simulink model "TEST_IPM_CPU2"  (R2019b)
settings: configuration reference "Configuration_CPU2" (kept outside this file)
libraries: c2837xDlib x2, c2000lib x1
settings Model: DataDictionary=TEST_IPM_LIB.sldd  Creator=Downstream  LastModifiedBy=Downstream
settings ConfigSetRef: SourceName=Configuration_CPU2

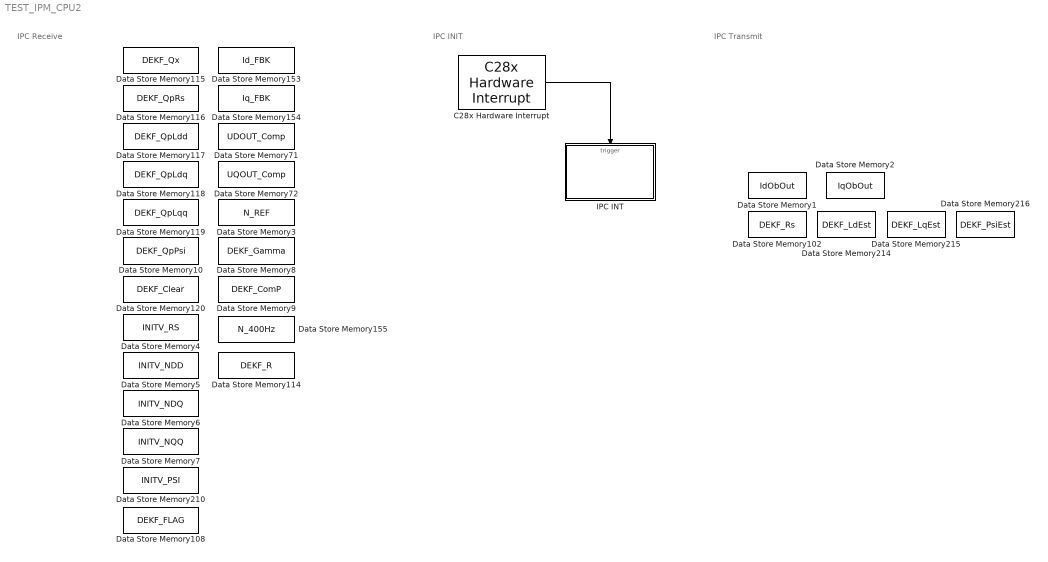
== system TEST_IPM_CPU2 ==
  note: IPC INIT
  note: IPC Receive
  note: IPC Transmit
  C28x Hardware Interrupt : c2000lib/Scheduling/C28x Hardware Interrupt  irqnumbers=[1]  pienumbers=[13]  irqpriorities=[4]  irqpreempts=[0]  showinput=off  dspchiptype=C280X
      settings: SourceProductName=Embedded Coder Support Package for Texas Instruments C2000 Processors  SourceProductBaseCode=TIC2000
  Data Store Memory1 : DataStoreMemory  DataStoreName=IdObOut  ReadBeforeWriteMsg=warning  WriteAfterWriteMsg=warning  WriteAfterReadMsg=warning  ShowAdditionalParam=off  OutDataTypeStr=single
      settings: RTWStateStorageClass=ExportedGlobal
  Data Store Memory10 : DataStoreMemory  DataStoreName=DEKF_QpPsi  ReadBeforeWriteMsg=warning  WriteAfterWriteMsg=warning  WriteAfterReadMsg=warning  InitialValue=0.047  ShowAdditionalParam=off  OutDataTypeStr=single
      settings: RTWStateStorageClass=ExportedGlobal
  Data Store Memory102 : DataStoreMemory  DataStoreName=DEKF_Rs  ReadBeforeWriteMsg=warning  WriteAfterWriteMsg=warning  WriteAfterReadMsg=warning  ShowAdditionalParam=off  OutDataTypeStr=single
      settings: RTWStateStorageClass=ExportedGlobal
  Data Store Memory108 : DataStoreMemory  DataStoreName=DEKF_FLAG  ReadBeforeWriteMsg=warning  WriteAfterWriteMsg=warning  WriteAfterReadMsg=warning  ShowAdditionalParam=off  OutDataTypeStr=uint16
      settings: RTWStateStorageClass=ExportedGlobal
  Data Store Memory114 : DataStoreMemory  DataStoreName=DEKF_R  ReadBeforeWriteMsg=warning  WriteAfterWriteMsg=warning  WriteAfterReadMsg=warning  ShowAdditionalParam=off  OutDataTypeStr=single
      settings: RTWStateStorageClass=ExportedGlobal
  Data Store Memory115 : DataStoreMemory  DataStoreName=DEKF_Qx  ReadBeforeWriteMsg=warning  WriteAfterWriteMsg=warning  WriteAfterReadMsg=warning  ShowAdditionalParam=off  OutDataTypeStr=single
      settings: RTWStateStorageClass=ExportedGlobal
  Data Store Memory116 : DataStoreMemory  DataStoreName=DEKF_QpRs  ReadBeforeWriteMsg=warning  WriteAfterWriteMsg=warning  WriteAfterReadMsg=warning  ShowAdditionalParam=off  OutDataTypeStr=single
      settings: RTWStateStorageClass=ExportedGlobal
  Data Store Memory117 : DataStoreMemory  DataStoreName=DEKF_QpLdd  ReadBeforeWriteMsg=warning  WriteAfterWriteMsg=warning  WriteAfterReadMsg=warning  ShowAdditionalParam=off  OutDataTypeStr=single
      settings: RTWStateStorageClass=ExportedGlobal
  Data Store Memory118 : DataStoreMemory  DataStoreName=DEKF_QpLdq  ReadBeforeWriteMsg=warning  WriteAfterWriteMsg=warning  WriteAfterReadMsg=warning  ShowAdditionalParam=off  OutDataTypeStr=single
      settings: RTWStateStorageClass=ExportedGlobal
  Data Store Memory119 : DataStoreMemory  DataStoreName=DEKF_QpLqq  ReadBeforeWriteMsg=warning  WriteAfterWriteMsg=warning  WriteAfterReadMsg=warning  ShowAdditionalParam=off  OutDataTypeStr=single
      settings: RTWStateStorageClass=ExportedGlobal
  Data Store Memory120 : DataStoreMemory  DataStoreName=DEKF_Clear  ReadBeforeWriteMsg=warning  WriteAfterWriteMsg=warning  WriteAfterReadMsg=warning  ShowAdditionalParam=off  OutDataTypeStr=uint16
      settings: RTWStateStorageClass=ExportedGlobal
  Data Store Memory153 : DataStoreMemory  DataStoreName=Id_FBK  ReadBeforeWriteMsg=warning  WriteAfterWriteMsg=warning  WriteAfterReadMsg=warning  ShowAdditionalParam=off  OutDataTypeStr=single
      settings: RTWStateStorageClass=ExportedGlobal
  Data Store Memory154 : DataStoreMemory  DataStoreName=Iq_FBK  ReadBeforeWriteMsg=warning  WriteAfterWriteMsg=warning  WriteAfterReadMsg=warning  ShowAdditionalParam=off  OutDataTypeStr=single
      settings: RTWStateStorageClass=ExportedGlobal
  Data Store Memory155 : DataStoreMemory  DataStoreName=N_400Hz  ReadBeforeWriteMsg=warning  WriteAfterWriteMsg=warning  WriteAfterReadMsg=warning  ShowAdditionalParam=off  OutDataTypeStr=single
      settings: RTWStateStorageClass=ExportedGlobal
  Data Store Memory2 : DataStoreMemory  DataStoreName=IqObOut  ReadBeforeWriteMsg=warning  WriteAfterWriteMsg=warning  WriteAfterReadMsg=warning  ShowAdditionalParam=off  OutDataTypeStr=single
      settings: RTWStateStorageClass=ExportedGlobal
  Data Store Memory210 : DataStoreMemory  DataStoreName=INITV_PSI  ReadBeforeWriteMsg=warning  WriteAfterWriteMsg=warning  WriteAfterReadMsg=warning  InitialValue=0.047  ShowAdditionalParam=off  OutDataTypeStr=single
      settings: RTWStateStorageClass=ExportedGlobal
  Data Store Memory214 : DataStoreMemory  DataStoreName=DEKF_LdEst  ReadBeforeWriteMsg=warning  WriteAfterWriteMsg=warning  WriteAfterReadMsg=warning  ShowAdditionalParam=off  OutDataTypeStr=single
      settings: RTWStateStorageClass=ExportedGlobal
  Data Store Memory215 : DataStoreMemory  DataStoreName=DEKF_LqEst  ReadBeforeWriteMsg=warning  WriteAfterWriteMsg=warning  WriteAfterReadMsg=warning  ShowAdditionalParam=off  OutDataTypeStr=single
      settings: RTWStateStorageClass=ExportedGlobal
  Data Store Memory216 : DataStoreMemory  DataStoreName=DEKF_PsiEst  ReadBeforeWriteMsg=warning  WriteAfterWriteMsg=warning  WriteAfterReadMsg=warning  ShowAdditionalParam=off  OutDataTypeStr=single
      settings: RTWStateStorageClass=ExportedGlobal
  Data Store Memory3 : DataStoreMemory  DataStoreName=N_REF  ReadBeforeWriteMsg=warning  WriteAfterWriteMsg=warning  WriteAfterReadMsg=warning  ShowAdditionalParam=off  OutDataTypeStr=single
      settings: RTWStateStorageClass=ExportedGlobal
  Data Store Memory4 : DataStoreMemory  DataStoreName=INITV_RS  ReadBeforeWriteMsg=warning  WriteAfterWriteMsg=warning  WriteAfterReadMsg=warning  InitialValue=0.93  ShowAdditionalParam=off  OutDataTypeStr=single
      settings: RTWStateStorageClass=ExportedGlobal
  Data Store Memory5 : DataStoreMemory  DataStoreName=INITV_NDD  ReadBeforeWriteMsg=warning  WriteAfterWriteMsg=warning  WriteAfterReadMsg=warning  InitialValue=1/2.7e-3  ShowAdditionalParam=off  OutDataTypeStr=single
      settings: RTWStateStorageClass=ExportedGlobal
  Data Store Memory6 : DataStoreMemory  DataStoreName=INITV_NDQ  ReadBeforeWriteMsg=warning  WriteAfterWriteMsg=warning  WriteAfterReadMsg=warning  ShowAdditionalParam=off  OutDataTypeStr=single
      settings: RTWStateStorageClass=ExportedGlobal
  Data Store Memory7 : DataStoreMemory  DataStoreName=INITV_NQQ  ReadBeforeWriteMsg=warning  WriteAfterWriteMsg=warning  WriteAfterReadMsg=warning  InitialValue=1/4.9e-3  ShowAdditionalParam=off  OutDataTypeStr=single
      settings: RTWStateStorageClass=ExportedGlobal
  Data Store Memory71 : DataStoreMemory  DataStoreName=UDOUT_Comp  ReadBeforeWriteMsg=warning  WriteAfterWriteMsg=warning  WriteAfterReadMsg=warning  ShowAdditionalParam=off  OutDataTypeStr=single
      settings: RTWStateStorageClass=ExportedGlobal
  Data Store Memory72 : DataStoreMemory  DataStoreName=UQOUT_Comp  ReadBeforeWriteMsg=warning  WriteAfterWriteMsg=warning  WriteAfterReadMsg=warning  ShowAdditionalParam=off  OutDataTypeStr=single
      settings: RTWStateStorageClass=ExportedGlobal
  Data Store Memory8 : DataStoreMemory  DataStoreName=DEKF_Gamma  ReadBeforeWriteMsg=warning  WriteAfterWriteMsg=warning  WriteAfterReadMsg=warning  ShowAdditionalParam=off  OutDataTypeStr=single
      settings: RTWStateStorageClass=ExportedGlobal
  Data Store Memory9 : DataStoreMemory  DataStoreName=DEKF_ComP  ReadBeforeWriteMsg=warning  WriteAfterWriteMsg=warning  WriteAfterReadMsg=warning  ShowAdditionalParam=off  OutDataTypeStr=single
      settings: RTWStateStorageClass=ExportedGlobal
  IPC INT : Subsystem  TreatAsAtomicUnit=on
  wires:
  C28x Hardware Interrupt/1 -> IPC INT/Trigger

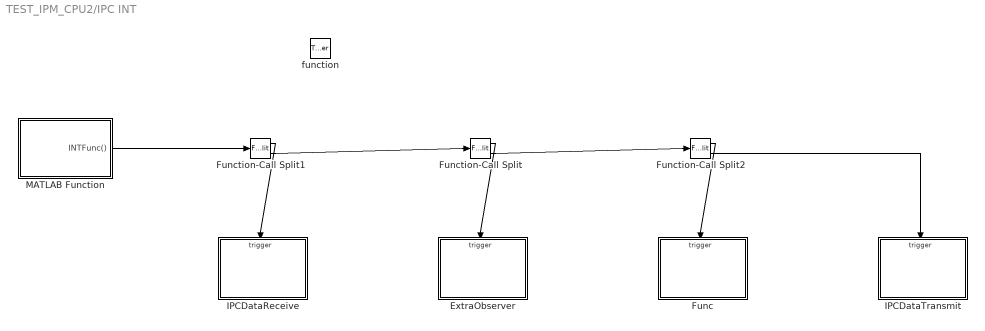
== system TEST_IPM_CPU2/IPC INT ==
  function : TriggerPort  TriggerType=function-call  VariantControl=Variant
  ExtraObserver : Subsystem
  Func : Subsystem
  Function-Call Split : FunctionCallSplit  NumOutputPorts=2
  Function-Call Split1 : FunctionCallSplit  NumOutputPorts=2
  Function-Call Split2 : FunctionCallSplit  NumOutputPorts=2
  IPCDataReceive : Subsystem
  IPCDataTransmit : Subsystem
  MATLAB Function : MATLAB Function  TreatAsAtomicUnit=on
  wires:
  MATLAB Function/1(INTFunc()) -> Function-Call Split1/1
  Function-Call Split1/1 -> IPCDataReceive/Trigger
  Function-Call Split/1 -> ExtraObserver/Trigger
  Function-Call Split1/2 -> Function-Call Split/1
  Function-Call Split/2 -> Function-Call Split2/1
  Function-Call Split2/2 -> IPCDataTransmit/Trigger
  Function-Call Split2/1 -> Func/Trigger

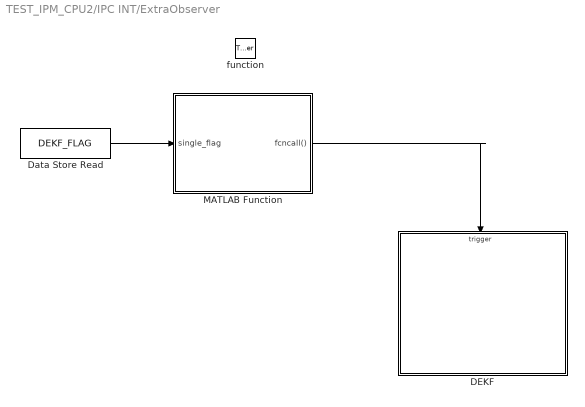
== system TEST_IPM_CPU2/IPC INT/ExtraObserver ==
  function : TriggerPort  TriggerType=function-call  VariantControl=Variant
  DEKF : Subsystem  TreatAsAtomicUnit=on
  Data Store Read : DataStoreRead  DataStoreName=DEKF_FLAG
  MATLAB Function : MATLAB Function  TreatAsAtomicUnit=on
  wires:
  Data Store Read/1 -> MATLAB Function/1(single_flag)
  MATLAB Function/1(fcncall()) -> DEKF/Trigger

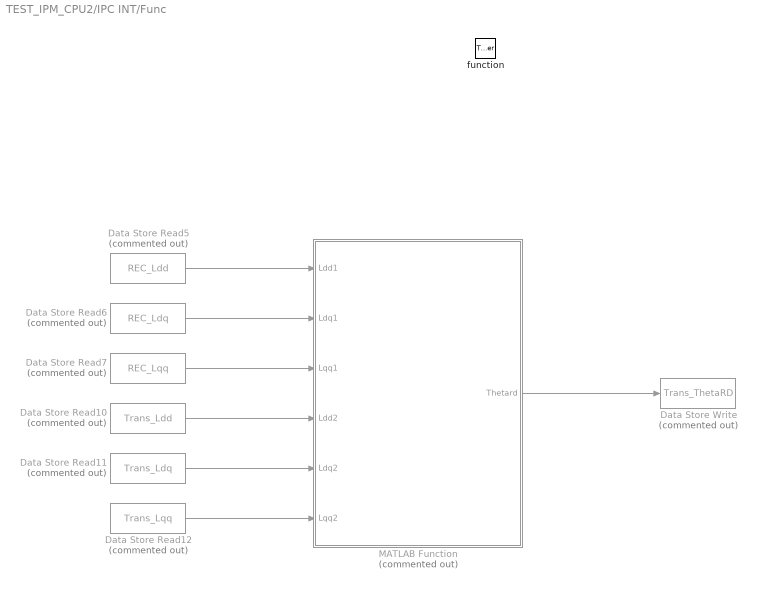
== system TEST_IPM_CPU2/IPC INT/Func ==
  function : TriggerPort  TriggerType=function-call  VariantControl=Variant
  Data Store Read10 : DataStoreRead  Commented=on  DataStoreName=Trans_Ldd
  Data Store Read11 : DataStoreRead  Commented=on  DataStoreName=Trans_Ldq
  Data Store Read12 : DataStoreRead  Commented=on  DataStoreName=Trans_Lqq
  Data Store Read5 : DataStoreRead  Commented=on  DataStoreName=REC_Ldd
  Data Store Read6 : DataStoreRead  Commented=on  DataStoreName=REC_Ldq
  Data Store Read7 : DataStoreRead  Commented=on  DataStoreName=REC_Lqq
  Data Store Write : DataStoreWrite  Commented=on  DataStoreName=Trans_ThetaRD
  MATLAB Function : MATLAB Function  Commented=on  TreatAsAtomicUnit=on
  wires:
  Data Store Read5/1 -> MATLAB Function/1(Ldd1)
  Data Store Read6/1 -> MATLAB Function/2(Ldq1)
  Data Store Read7/1 -> MATLAB Function/3(Lqq1)
  Data Store Read10/1 -> MATLAB Function/4(Ldd2)
  Data Store Read11/1 -> MATLAB Function/5(Ldq2)
  Data Store Read12/1 -> MATLAB Function/6(Lqq2)
  MATLAB Function/1(Thetard) -> Data Store Write/1

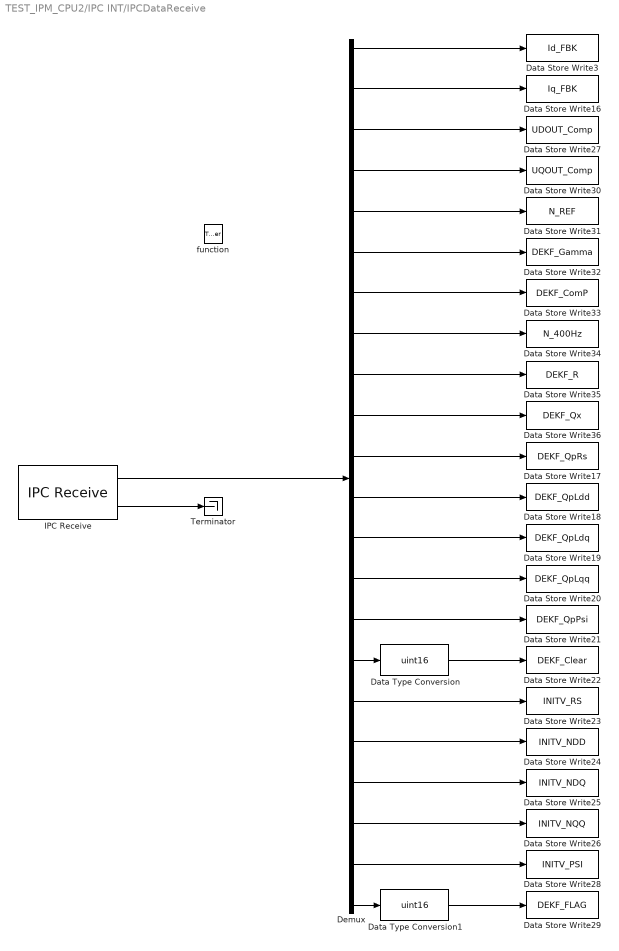
== system TEST_IPM_CPU2/IPC INT/IPCDataReceive ==
  function : TriggerPort  TriggerType=function-call  VariantControl=Variant
  Data Store Write16 : DataStoreWrite  DataStoreName=Iq_FBK
  Data Store Write17 : DataStoreWrite  DataStoreName=DEKF_QpRs
  Data Store Write18 : DataStoreWrite  DataStoreName=DEKF_QpLdd
  Data Store Write19 : DataStoreWrite  DataStoreName=DEKF_QpLdq
  Data Store Write20 : DataStoreWrite  DataStoreName=DEKF_QpLqq
  Data Store Write21 : DataStoreWrite  DataStoreName=DEKF_QpPsi
  Data Store Write22 : DataStoreWrite  DataStoreName=DEKF_Clear
  Data Store Write23 : DataStoreWrite  DataStoreName=INITV_RS
  Data Store Write24 : DataStoreWrite  DataStoreName=INITV_NDD
  Data Store Write25 : DataStoreWrite  DataStoreName=INITV_NDQ
  Data Store Write26 : DataStoreWrite  DataStoreName=INITV_NQQ
  Data Store Write27 : DataStoreWrite  DataStoreName=UDOUT_Comp
  Data Store Write28 : DataStoreWrite  DataStoreName=INITV_PSI
  Data Store Write29 : DataStoreWrite  DataStoreName=DEKF_FLAG
  Data Store Write3 : DataStoreWrite  DataStoreName=Id_FBK
  Data Store Write30 : DataStoreWrite  DataStoreName=UQOUT_Comp
  Data Store Write31 : DataStoreWrite  DataStoreName=N_REF
  Data Store Write32 : DataStoreWrite  DataStoreName=DEKF_Gamma
  Data Store Write33 : DataStoreWrite  DataStoreName=DEKF_ComP
  Data Store Write34 : DataStoreWrite  DataStoreName=N_400Hz
  Data Store Write35 : DataStoreWrite  DataStoreName=DEKF_R
  Data Store Write36 : DataStoreWrite  DataStoreName=DEKF_Qx
  Data Type Conversion : DataTypeConversion  OutDataTypeStr=uint16
  Data Type Conversion1 : DataTypeConversion  OutDataTypeStr=uint16
  Demux : Demux  Outputs=22
  IPC Receive : c2837xDlib/IPC Receive  SelectChannel=0  DataType=single  DataLength=22  EnableBlocking=off  SampleTime=-1
      settings: SourceProductName=Embedded Coder Support Package for Texas Instruments C2000 Processors  SourceProductBaseCode=TIC2000
  Terminator : Terminator
  wires:
  IPC Receive/1 -> Demux/1
  IPC Receive/2 -> Terminator/1
  Demux/1 -> Data Store Write3/1
  Demux/2 -> Data Store Write16/1
  Demux/3 -> Data Store Write27/1
  Demux/4 -> Data Store Write30/1
  Demux/5 -> Data Store Write31/1
  Demux/6 -> Data Store Write32/1
  Demux/7 -> Data Store Write33/1
  Demux/8 -> Data Store Write34/1
  Demux/9 -> Data Store Write35/1
  Demux/10 -> Data Store Write36/1
  Demux/11 -> Data Store Write17/1
  Demux/12 -> Data Store Write18/1
  Demux/13 -> Data Store Write19/1
  Demux/14 -> Data Store Write20/1
  Demux/15 -> Data Store Write21/1
  Demux/16 -> Data Type Conversion/1
  Demux/17 -> Data Store Write23/1
  Demux/18 -> Data Store Write24/1
  Demux/19 -> Data Store Write25/1
  Demux/20 -> Data Store Write26/1
  Demux/21 -> Data Store Write28/1
  Demux/22 -> Data Type Conversion1/1
  Data Type Conversion/1 -> Data Store Write22/1
  Data Type Conversion1/1 -> Data Store Write29/1

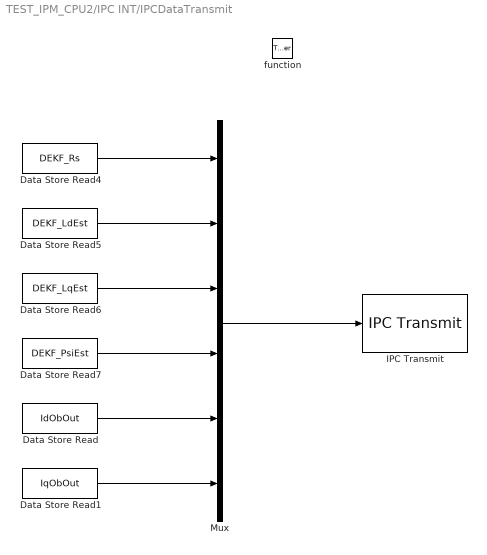
== system TEST_IPM_CPU2/IPC INT/IPCDataTransmit ==
  function : TriggerPort  TriggerType=function-call  VariantControl=Variant
  Data Store Read : DataStoreRead  DataStoreName=IdObOut
  Data Store Read1 : DataStoreRead  DataStoreName=IqObOut
  Data Store Read4 : DataStoreRead  DataStoreName=DEKF_Rs
  Data Store Read5 : DataStoreRead  DataStoreName=DEKF_LdEst
  Data Store Read6 : DataStoreRead  DataStoreName=DEKF_LqEst
  Data Store Read7 : DataStoreRead  DataStoreName=DEKF_PsiEst
  IPC Transmit : c2837xDlib/IPC Transmit  SelectChannel=1  EnableBlocking=off
      settings: SourceProductName=Embedded Coder Support Package for Texas Instruments C2000 Processors  SourceProductBaseCode=TIC2000
  Mux : Mux  Inputs=6
  wires:
  Mux/1 -> IPC Transmit/1
  Data Store Read4/1 -> Mux/1
  Data Store Read5/1 -> Mux/2
  Data Store Read6/1 -> Mux/3
  Data Store Read7/1 -> Mux/4
  Data Store Read/1 -> Mux/5
  Data Store Read1/1 -> Mux/6

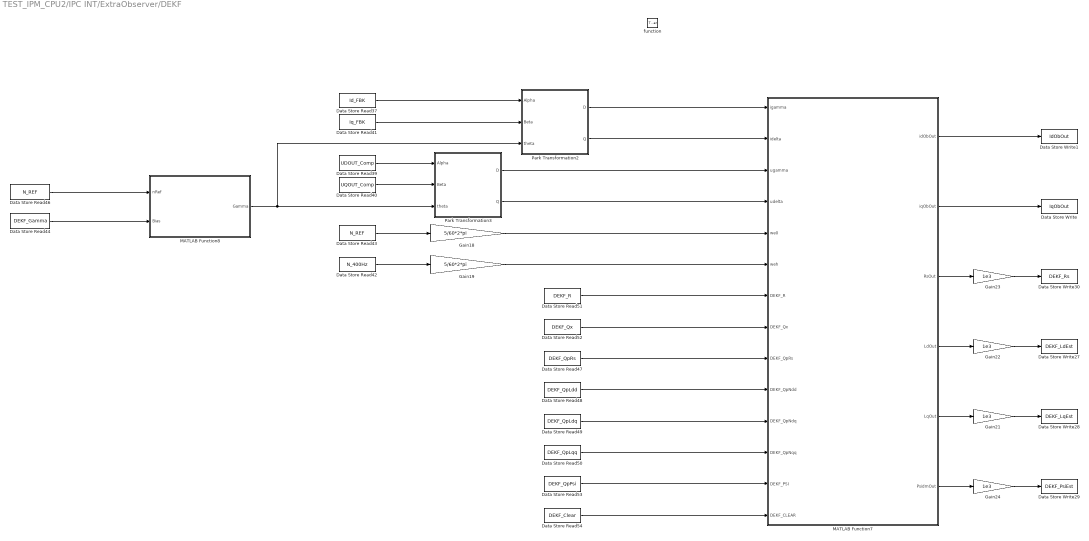
== system TEST_IPM_CPU2/IPC INT/ExtraObserver/DEKF ==
  function : TriggerPort  TriggerType=function-call  VariantControl=Variant
  Data Store Read37 : DataStoreRead  DataStoreName=Id_FBK
  Data Store Read39 : DataStoreRead  DataStoreName=UDOUT_Comp
  Data Store Read40 : DataStoreRead  DataStoreName=UQOUT_Comp
  Data Store Read41 : DataStoreRead  DataStoreName=Iq_FBK
  Data Store Read42 : DataStoreRead  DataStoreName=N_400Hz
  Data Store Read43 : DataStoreRead  DataStoreName=N_REF
  Data Store Read44 : DataStoreRead  DataStoreName=DEKF_Gamma
  Data Store Read46 : DataStoreRead  DataStoreName=N_REF
  Data Store Read47 : DataStoreRead  DataStoreName=DEKF_QpRs
  Data Store Read48 : DataStoreRead  DataStoreName=DEKF_QpLdd
  Data Store Read49 : DataStoreRead  DataStoreName=DEKF_QpLdq
  Data Store Read50 : DataStoreRead  DataStoreName=DEKF_QpLqq
  Data Store Read51 : DataStoreRead  DataStoreName=DEKF_R
  Data Store Read52 : DataStoreRead  DataStoreName=DEKF_Qx
  Data Store Read53 : DataStoreRead  DataStoreName=DEKF_QpPsi
  Data Store Read54 : DataStoreRead  DataStoreName=DEKF_Clear
  Data Store Write : DataStoreWrite  DataStoreName=IqObOut
  Data Store Write1 : DataStoreWrite  DataStoreName=IdObOut
  Data Store Write27 : DataStoreWrite  DataStoreName=DEKF_LdEst
  Data Store Write28 : DataStoreWrite  DataStoreName=DEKF_LqEst
  Data Store Write29 : DataStoreWrite  DataStoreName=DEKF_PsiEst
  Data Store Write30 : DataStoreWrite  DataStoreName=DEKF_Rs
  Gain18 : Gain  Gain=5/60*2*pi
  Gain19 : Gain  Gain=5/60*2*pi
  Gain{21..24} (4 alike) : Gain  Gain=1e3
  MATLAB Function7 : MATLAB Function  TreatAsAtomicUnit=on
  MATLAB Function8 : MATLAB Function  TreatAsAtomicUnit=on
  Park Transformation2 : Subsystem
  Park Transformation3 : Subsystem
  wires:
  Data Store Read49/1 -> MATLAB Function7/11(DEKF_QpNdq)
  Data Store Read37/1 -> Park Transformation2/1(Alpha)
  Data Store Read41/1 -> Park Transformation2/2(Beta)
  Data Store Read40/1 -> Park Transformation3/2(Beta)
  Gain18/1 -> MATLAB Function7/5(we0)
  MATLAB Function8/1(Gamma) -> Park Transformation3/3(theta), Park Transformation2/3(theta)
  Park Transformation2/1(D) -> MATLAB Function7/1(igamma)
  Data Store Read39/1 -> Park Transformation3/1(Alpha)
  Park Transformation3/2(Q) -> MATLAB Function7/4(udelta)
  Park Transformation3/1(D) -> MATLAB Function7/3(ugamma)
  Data Store Read52/1 -> MATLAB Function7/8(DEKF_Qx)
  Data Store Read53/1 -> MATLAB Function7/13(DEKF_PSI)
  Park Transformation2/2(Q) -> MATLAB Function7/2(idelta)
  Data Store Read51/1 -> MATLAB Function7/7(DEKF_R)
  Gain24/1 -> Data Store Write29/1
  Data Store Read54/1 -> MATLAB Function7/14(DEKF_CLEAR)
  MATLAB Function7/5(LqOut) -> Gain21/1
  MATLAB Function7/4(LdOut) -> Gain22/1
  Gain23/1 -> Data Store Write30/1
  Data Store Read43/1 -> Gain18/1
  Data Store Read47/1 -> MATLAB Function7/9(DEKF_QpRs)
  Data Store Read48/1 -> MATLAB Function7/10(DEKF_QpNdd)
  Gain22/1 -> Data Store Write27/1
  MATLAB Function7/3(RsOut) -> Gain23/1
  Data Store Read50/1 -> MATLAB Function7/12(DEKF_QpNqq)
  Gain19/1 -> MATLAB Function7/6(weh)
  Gain21/1 -> Data Store Write28/1
  MATLAB Function7/6(PsidmOut) -> Gain24/1
  Data Store Read42/1 -> Gain19/1
  Data Store Read44/1 -> MATLAB Function8/2(Bias)
  Data Store Read46/1 -> MATLAB Function8/1(nRef)
  MATLAB Function7/2(iqObOut) -> Data Store Write/1
  MATLAB Function7/1(idObOut) -> Data Store Write1/1

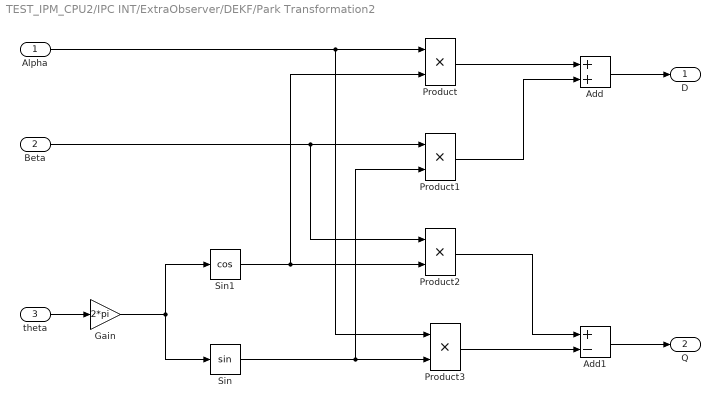
== system TEST_IPM_CPU2/IPC INT/ExtraObserver/DEKF/Park Transformation2 ==
  Alpha : Inport
  Beta : Inport  Port=2
  theta : Inport  Port=3
  Add : Sum
  Add1 : Sum  Inputs=+-
  Gain : Gain  Gain=2*pi
  Product{,1..3} (4 alike) : Product
  Sin : Trigonometry  OutputSignalType=real
  Sin1 : Trigonometry  Operator=cos  OutputSignalType=real
  D : Outport
  Q : Outport  Port=2
  wires:
  Product/1 -> Add/1
  Sin/1 -> Product3/2, Product1/2
  Product1/1 -> Add/2
  Add1/1 -> Q/1
  Sin1/1 -> Product2/2, Product/2
  Product2/1 -> Add1/1
  Alpha/1 -> Product3/1, Product/1
  Beta/1 -> Product2/1, Product1/1
  Product3/1 -> Add1/2
  Add/1 -> D/1
  theta/1 -> Gain/1
  Gain/1 -> Sin/1, Sin1/1

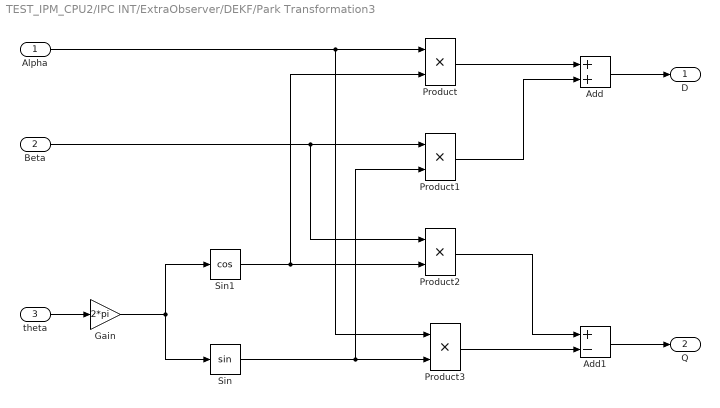
== system TEST_IPM_CPU2/IPC INT/ExtraObserver/DEKF/Park Transformation3 ==
  Alpha : Inport
  Beta : Inport  Port=2
  theta : Inport  Port=3
  Add : Sum
  Add1 : Sum  Inputs=+-
  Gain : Gain  Gain=2*pi
  Product{,1..3} (4 alike) : Product
  Sin : Trigonometry  OutputSignalType=real
  Sin1 : Trigonometry  Operator=cos  OutputSignalType=real
  D : Outport
  Q : Outport  Port=2
  wires:
  Gain/1 -> Sin1/1, Sin/1
  theta/1 -> Gain/1
  Add/1 -> D/1
  Product3/1 -> Add1/2
  Beta/1 -> Product1/1, Product2/1
  Alpha/1 -> Product/1, Product3/1
  Product2/1 -> Add1/1
  Sin1/1 -> Product/2, Product2/2
  Add1/1 -> Q/1
  Product1/1 -> Add/2
  Sin/1 -> Product1/2, Product3/2
  Product/1 -> Add/1

== matlab function TEST_IPM_CPU2/IPC INT/ExtraObserver/MATLAB Function ==
  data: single_flag input
  events: fcncall output FUNCTION_CALL_EVENT
function DEKF_FUNC(single_flag)
if (single_flag >= single(0.5))
    fcncall();
end

== matlab function TEST_IPM_CPU2/IPC INT/MATLAB Function ==
  events: INTFunc output FUNCTION_CALL_EVENT
function START
INTFunc();
end

== matlab function TEST_IPM_CPU2/IPC INT/Func/MATLAB Function ==
  data: Ldd1 input; Thetard output; Ldq1 input; Lqq1 input; Ldd2 input; Ldq2 input; Lqq2 input
function Thetard = ThetaError(Ldd1,Ldq1,Lqq1,Ldd2,Ldq2,Lqq2)
temp1 = (Ldd2 - Lqq2) - single(2) * Ldq1;
temp2 = (Ldd1 - Lqq1) + single(2) * Ldq2;
Thetard = single(0.5) * atan2(temp1,temp2) * single(57.2958);

== matlab function TEST_IPM_CPU2/IPC INT/ExtraObserver/DEKF/MATLAB Function7 ==
  data: idObOut output; iqObOut output; igamma input; RsOut output; idelta input; ugamma input; udelta input; we0 input; weh input; INITV_RS data_store_memory; INITV_NDD data_store_memory; INITV_NDQ data_store_memory; INITV_NQQ data_store_memory; INITV_PSI data_store_memory; DEKF_R input; DEKF_Qx input; DEKF_QpRs input; DEKF_QpNdd input; DEKF_QpNdq input; DEKF_QpNqq input; DEKF_PSI input; DEKF_CLEAR input; LdOut output; LqOut output; PsidmOut output
function [idObOut,iqObOut,RsOut,LdOut,LqOut,PsidmOut] = DEKF_ParamObSensorless(igamma,idelta,ugamma,udelta,we0,weh,DEKF_R,DEKF_Qx,DEKF_QpRs,DEKF_QpNdd,DEKF_QpNdq,DEKF_QpNqq,DEKF_PSI,DEKF_CLEAR)
global INITV_RS INITV_NDD INITV_NDQ INITV_NQQ INITV_PSI

persistent hat_x hat_param P_hat_x P_hat_param;
persistent difx_difparam K_xk_1 difH_difparam;
if isempty(hat_x)
    hat_x = single([0;0;]);
    hat_param = single([INITV_RS;INITV_NDD;INITV_NDQ;INITV_NQQ;INITV_PSI;]);
    P_hat_x = single(zeros(2));
    P_hat_param = single(zeros(5));
    
    difx_difparam = single(zeros(2,5));
    K_xk_1 = single(zeros(2));
    difH_difparam = single(zeros(2,5));
end
u = [ugamma;udelta;];
i = [igamma;idelta;];
Tsim = single(1e-4);
Qx = single([DEKF_Qx,0;0,DEKF_Qx;]);
Qp = single(diag([DEKF_QpRs DEKF_QpNdd DEKF_QpNdq DEKF_QpNqq DEKF_PSI]));
R = single([DEKF_R,0;0,DEKF_R;]);
J = single([0,-1;1,0]);

%Step1:Param Prior Estimation

param_PE = hat_param;

P_param_PE = P_hat_param + Qp;

%Step2: State Prior Estimation

Rs = param_PE(1);
Ngg = param_PE(2); Ngd = param_PE(3); Ndd = param_PE(4);
Psidm = param_PE(5);
we = we0 + weh;
N = [Ngg Ngd;Ngd Ndd;];
A = (Rs * N + we * J);
tilde_theta = 1/2 * atan(-2 * Ngd / (Ndd - Ngg));
dot_x = u - A * hat_x - we * J * Psidm * [cos(tilde_theta);sin(tilde_theta);];
x_PE = hat_x + dot_x * Tsim;

A_dis = eye(2) - A * Tsim;
P_x_PE = A_dis * P_hat_x * A_dis' + Qx;

%step3: State Kalman Gain
K_xk = P_x_PE * N' * (N * P_x_PE * N' + R)^-1;
P_hat_x = (eye(2) - K_xk * N) * P_x_PE;

%Step4: Param Kalman Gain
difhat_x_difparam = difx_difparam - K_xk_1 * difH_difparam;

TempA = we * Psidm * 1/2 * 1/(1 + (-2 * Ngd / (Ndd - Ngg))^2) * 1 / ((Ndd - Ngg)^2);
TempCOS = TempA * cos(tilde_theta); TempSIN = TempA * sin(tilde_theta);
C1 = TempCOS * single(-1);              C2 = TempSIN * single(-1);
C3 = TempCOS * single(2) * (Ndd - Ngg); C4 = TempSIN * single(2) * (Ndd - Ngg);
C5 = TempCOS * single( 1);              C6 = TempSIN * single( 1);

difG_difparam     = -Tsim * [Ngg * hat_x(1) + Ngd * hat_x(2), Rs * hat_x(1) + C1, Rs * hat_x(2) + C3, 0 + C5            , -we * sin(tilde_theta);...
                             Ngd * hat_x(1) + Ndd * hat_x(2), 0             + C2, Rs * hat_x(1) + C4, Rs * hat_x(2) + C6,  we * cos(tilde_theta);];
difG_difparam = difG_difparam + A_dis * difhat_x_difparam;
H_pk = [0, hat_x(1), hat_x(2), 0       , 0;...
        0, 0       , hat_x(1), hat_x(2), 0;];
H_pk = H_pk + N * difG_difparam;

K_pk = P_param_PE * H_pk' * (H_pk * P_param_PE * H_pk' + R)^-1;
P_hat_param = (eye(5) - K_pk * H_pk) * P_param_PE;
%step5: State & Param Prediction
hat_x = x_PE + K_xk * (i - N * x_PE);
hat_param = param_PE + K_pk * (i - N * x_PE);

if(hat_param(1) > single(2.0))
    hat_param(1) = single(2.0);
elseif(hat_param(1) < single(0.2))
    hat_param(1) = single(0.2);
end

if(hat_param(2) > single(3.7e3))
    hat_param(2) = single(3.7e3);
elseif(hat_param(2) < single(3.7e1))
    hat_param(2) = single(3.7e1);
end


if(hat_param(3) > single(3.7e2))
    hat_param(3) = single(3.7e2);
elseif(hat_param(3) < -single(3.7e2))
    hat_param(3) = -single(3.7e2);
end


if(hat_param(4) > single(2.0e3))
    hat_param(4) = single(2.0e3);
elseif(hat_param(4) < single(2.0e1))
    hat_param(4) = single(2.0e1);
end

if(hat_param(5) > single(0.1))
    hat_param(5) = single(0.1);
elseif(hat_param(5) < single(0.024))
    hat_param(5) = single(0.024);
end

%Step6: Update the parameter kalman gain
difx_difparam = difG_difparam;
K_xk_1 = K_xk;
difH_difparam = H_pk;

if(DEKF_CLEAR > single(0.5))
%     hat_x = single([0;0;]);
    hat_param = single([INITV_RS;INITV_NDD;INITV_NDQ;INITV_NQQ;INITV_PSI;]);
    NOut = [hat_param(2) hat_param(3);hat_param(3) hat_param(4);];
    hat_x = NOut * i;
    P_hat_x = single(zeros(2));
    P_hat_param = single(zeros(5));
    
    difx_difparam = single(zeros(2,5));
    K_xk_1 = single(zeros(2));
    difH_difparam = single(zeros(2,5));
end
P =     [cos(tilde_theta) sin(tilde_theta);-sin(tilde_theta) cos(tilde_theta);];
P_inv = [cos(tilde_theta) -sin(tilde_theta);sin(tilde_theta) cos(tilde_theta);];
NOut = [hat_param(2) hat_param(3);hat_param(3) hat_param(4);];
iObOut = NOut * hat_x;
idObOut = iObOut(1);
iqObOut = iObOut(2);
LOut = P_inv * (NOut^-1) * P;
RsOut = hat_param(1);
LdOut = LOut(1,1); LqOut = LOut(2,2);
PsidmOut = hat_param(5);

== matlab function TEST_IPM_CPU2/IPC INT/ExtraObserver/DEKF/MATLAB Function8 ==
  data: nRef input; Gamma output; Bias input
function Gamma = GammaComP(nRef,Bias)

% Gamma = single(5.819e-6) * nRef + Bias;
Gamma = Bias;
